simulink model "FMCWSim"  (R2021b)
settings: Solver=VariableStepAuto  StartTime=0.0  StopTime=stop_time  RelTol=1e-3
values from neighbouring files (symbols this model uses):
  num_samples_in_sampling_period = obj.ADC_Samples    [Radar.m]
  num_samples_prior_to_sample_period = int32((obj.ADC_ValidStartTime_us + obj.IdleTime_us) *                 obj.ADC_SampleRate_MSps)    [Radar.m]
  simulator = Simulator_revB()    [compute_sensed_targets.m]    (also in compute_sensed_values.m)
undefined symbols (not defined in the file or in its folder): designMultirateFIR, magnitude, physconst
libraries: phaseddetectlib x5, phasedenvlib x4, hdlsllib x4, simulink x2, phasedtxrxlib x2, phasedwavlib x1, dspswit3 x1, radarlib x1, dspmlti4 x1
settings Model: SimulationMode=accelerator  Creator=David  LastModifiedBy=David

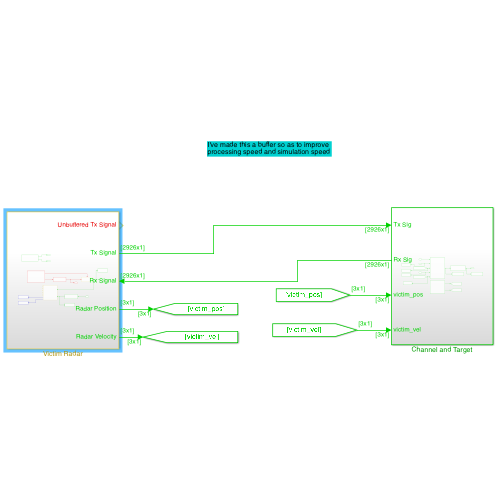
[thumbnail: Simulink's stored preview of the top-level diagram]
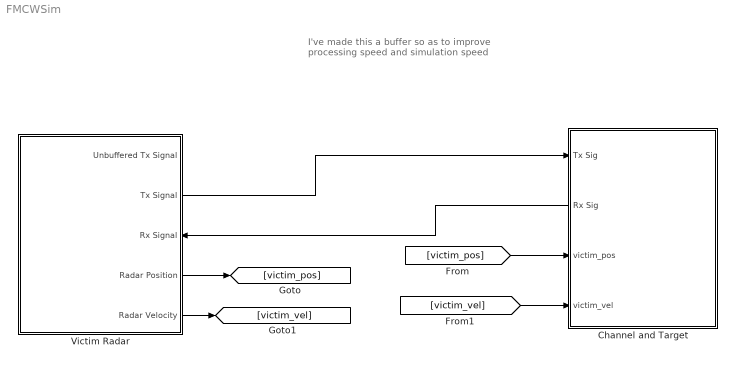
== system FMCWSim ==
  note: I've made this a buffer so as to improve
      | processing speed and simulation speed
  Channel and Target : Subsystem
      settings: PortSchema="{\"entries\":[{\"content\":{\"sides\":[{\"content\":{\"connectorIds\":[\"In1\",\"Out1\",\"In2\",\"In3\"]},\"type\":\"ConnectorPlacement.EquallySpacedRectSide\",\"uuid\":\"8c997438-cd57-4b9a-9eea-b04952771858\"},{\"content\":{\"connectorIds\":[],\"side\":\"RIGHT\"},\"type\":\"ConnectorPlacement.EquallySpacedRectSide\",\"uuid\":\"a5c22adb-228f-478b-86ad-e927dc02fa6c\"},{\"content\":{\"connectorIds\":[],\"side\":\"TOP\"},\"type\":\"ConnectorPlacement.EquallySpacedRectSide\",\"uuid\":\"b1cfcadd-6889-4e9e-8c43-7e76de170b82\"}]},\"type\":\"ConnectorPlacement.EquallySpacedConnector\",\"uuid\":\"fd8de1ec-06fb-4ea8-b936-70a4a20a8787\"}],\"packageUris\":[\"http://schema.mathworks.com/mf0/Connector/R2020b\"],\"version\":\"1.0\"}"
  Victim Radar : Subsystem
      settings: PortSchema="{\"entries\":[{\"content\":{\"sides\":[{\"content\":{\"connectorIds\":[]},\"type\":\"ConnectorPlacement.EquallySpacedRectSide\",\"uuid\":\"d1da3d36-0806-43d7-8452-bab3645a751c\"},{\"content\":{\"connectorIds\":[\"Out1\",\"Out2\",\"In1\",\"Out3\",\"Out4\"],\"side\":\"RIGHT\"},\"type\":\"ConnectorPlacement.EquallySpacedRectSide\",\"uuid\":\"352ec7eb-fc0a-43de-8b0c-663d6e923176\"},{\"content\":{\"connectorIds\":[],\"side\":\"TOP\"},\"type\":\"ConnectorPlacement.EquallySpacedRectSide\",\"uuid\":\"55e1007f-228b-4090-badb-c8b9047c2b51\"}]},\"type\":\"ConnectorPlacement.EquallySpacedConnector\",\"uuid\":\"2018d0fb-49bb-41d2-bc14-1588bf842768\"}],\"packageUris\":[\"http://schema.mathworks.com/mf0/Connector/R2020b\"],\"version\":\"1.0\"}"
  wires:
  [victim_pos] -> Channel and Target/2(victim_pos)
  [victim_vel] -> Channel and Target/3(victim_vel)
  Victim Radar/2(Tx Signal) -> Channel and Target/1(Tx Sig)
  Victim Radar/4(Radar Velocity) -> [victim_vel]
  Victim Radar/3(Radar Position) -> [victim_pos]
  Channel and Target/1(Rx Sig) -> Victim Radar/1(Rx Signal)

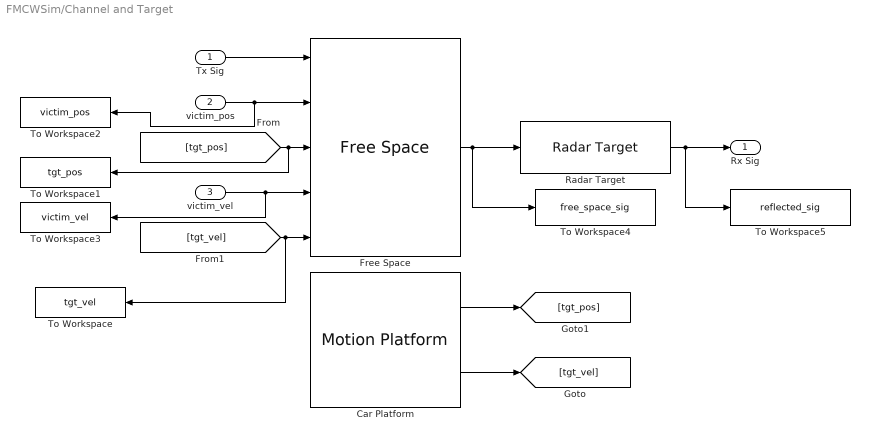
== system FMCWSim/Channel and Target ==
  Tx Sig : Inport
  victim_pos : Inport  Port=2
  victim_vel : Inport  Port=3
  Car Platform : phasedenvlib/Motion Platform  MotionModel=Velocity  InitialPosition=simulator.SimulatedTarget.position_m  InitialVelocity=[ 0; 0; 0 ]  VelocitySource=Property  Velocity=simulator.SimulatedTarget.velocity_meters_per_s  AccelerationSource=Property  Acceleration=[0;0;0]  CustomTrajectory=[ 0, 0, 0, 0, 0, 0, 0; 1, 0, 0, 0, 0, 0, 0 ]  ScanMode=None  InitialScanAngle=0  AzimuthSpan=[ -60, 60 ]  AzimuthScanRate=10  InitialOrientationAxes=eye( 3 )  OrientationAxesOutputPort=off  ElapsedTimeSource=Auto  SampleRateFromInputCheckbox=on  SampleRate=1e6  SimulateUsing=Interpreted execution
      settings: SourceProductBaseCode=AR
  Free Space : phasedenvlib/Free Space  PropagationSpeed=physconst( 'LightSpeed' )  OperatingFrequency=simulator.SimulatedTarget.operating_frequency_Hz  TwoWayPropagation=on  SampleRateFromInputCheckbox=off  SampleRate=simulator.Victim.FMCW_sampling_rate_Hz  MaximumDistanceSource=Property  MaximumDistance=1e3  MaximumNumInputSamplesSource=Auto  MaximumNumInputSamples=1000  SimulateUsing=Interpreted execution
      settings: SourceProductBaseCode=AR
  Radar Target : phasedenvlib/Radar Target  EnablePolarization=off  Mode=Monostatic  MeanRCSSource=Property  ScatteringMatrixSource=Property  MeanRCS=simulator.SimulatedTarget.rcs_sq_meters  ScatteringMatrix=eye( 2 )  Model=Nonfluctuating  PropagationSpeed=physconst( 'LightSpeed' )  OperatingFrequency=simulator.SimulatedTarget.operating_frequency_Hz  SeedSource=Auto  Seed=0  SimulateUsing=Interpreted execution
      settings: SourceProductBaseCode=AR
  To Workspace : ToWorkspace  VariableName=tgt_vel  SampleTime=-1
      settings: MaxDataPoints=2
  To Workspace1 : ToWorkspace  VariableName=tgt_pos  SampleTime=-1
      settings: MaxDataPoints=2
  To Workspace2 : ToWorkspace  VariableName=victim_pos  SampleTime=-1
      settings: MaxDataPoints=2
  To Workspace3 : ToWorkspace  VariableName=victim_vel  SampleTime=-1
      settings: MaxDataPoints=2
  To Workspace4 : ToWorkspace  VariableName=free_space_sig  SampleTime=-1
      settings: MaxDataPoints=2
  To Workspace5 : ToWorkspace  VariableName=reflected_sig  SampleTime=-1
      settings: MaxDataPoints=2
  Rx Sig : Outport
  wires:
  Tx Sig/1 -> Free Space/1
  victim_pos/1 -> To Workspace2/1, Free Space/2
  victim_vel/1 -> To Workspace3/1, Free Space/4
  [tgt_vel] -> To Workspace/1, Free Space/5
  [tgt_pos] -> To Workspace1/1, Free Space/3
  Car Platform/1 -> [tgt_pos]
  Car Platform/2 -> [tgt_vel]
  Radar Target/1 -> To Workspace5/1, Rx Sig/1
  Free Space/1 -> To Workspace4/1, Radar Target/1

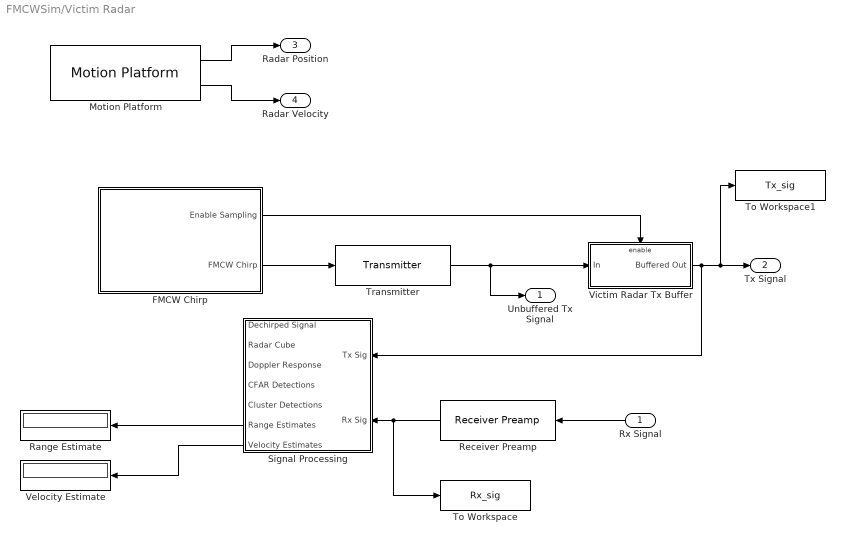
== system FMCWSim/Victim Radar ==
  Rx Signal : Inport
  FMCW Chirp : Subsystem
  Motion Platform : phasedenvlib/Motion Platform  MotionModel=Velocity  InitialPosition=simulator.Victim.position_m  InitialVelocity=[ 0; 0; 0 ]  VelocitySource=Property  Velocity=simulator.Victim.velocity_m_per_s  AccelerationSource=Property  Acceleration=[0;0;0]  CustomTrajectory=[ 0, 0, 0, 0, 0, 0, 0; 1, 0, 0, 0, 0, 0, 0 ]  ScanMode=None  InitialScanAngle=0  AzimuthSpan=[ -60, 60 ]  AzimuthScanRate=10  InitialOrientationAxes=eye( 3 )  OrientationAxesOutputPort=off  ElapsedTimeSource=Auto  SampleRateFromInputCheckbox=on  SampleRate=1e6  SimulateUsing=Interpreted execution
      settings: SourceProductBaseCode=AR
  Range Estimate : Display
  Receiver Preamp : phasedtxrxlib/Receiver Preamp  Gain=simulator.Victim.rx_gain_dB  LossFactor=0  NoiseMethod=Noise temperature  NoiseFigure=simulator.Victim.rx_nf_dB  ReferenceTemperature=290  SampleRateFromInputCheckbox=off  SampleRate=simulator.Victim.FMCW_sampling_rate_Hz  NoisePower=0  EnableInputPort=off  PhaseNoiseInputPort=off  SeedSource=Auto  Seed=0  SimulateUsing=Interpreted execution
      settings: SourceProductBaseCode=AR
  Signal Processing : Subsystem
  To Workspace : ToWorkspace  VariableName=Rx_sig  SampleTime=-1
      settings: MaxDataPoints=2
  To Workspace1 : ToWorkspace  VariableName=Tx_sig  SampleTime=-1
      settings: MaxDataPoints=2
  Transmitter : phasedtxrxlib/Transmitter  PeakPower=simulator.Victim.tx_power_W  Gain=simulator.Victim.tx_gain_dB  LossFactor=0  InUseOutputPort=off  CoherentOnTransmit=on  PhaseNoiseOutputPort=off  SeedSource=Auto  Seed=0  SimulateUsing=Interpreted execution
      settings: SourceProductBaseCode=AR
  Velocity Estimate : Display
  Victim Radar Tx Buffer : Subsystem  TreatAsAtomicUnit=on
  Unbuffered Tx Signal : Outport
  Tx Signal : Outport  Port=2
  Radar Position : Outport  Port=3
  Radar Velocity : Outport  Port=4
  wires:
  Rx Signal/1 -> Receiver Preamp/1
  Receiver Preamp/1 -> To Workspace/1, Signal Processing/2(Rx Sig)
  Signal Processing/6(Range Estimates) -> Range Estimate/1
  Signal Processing/7(Velocity Estimates) -> Velocity Estimate/1
  Motion Platform/2 -> Radar Velocity/1
  Motion Platform/1 -> Radar Position/1
  FMCW Chirp/2(FMCW Chirp) -> Transmitter/1
  FMCW Chirp/1(Enable Sampling) -> Victim Radar Tx Buffer/Enable
  Transmitter/1 -> Unbuffered Tx Signal/1, Victim Radar Tx Buffer/1(In)
  Victim Radar Tx Buffer/1(Buffered Out) -> To Workspace1/1, Tx Signal/1, Signal Processing/1(Tx Sig)

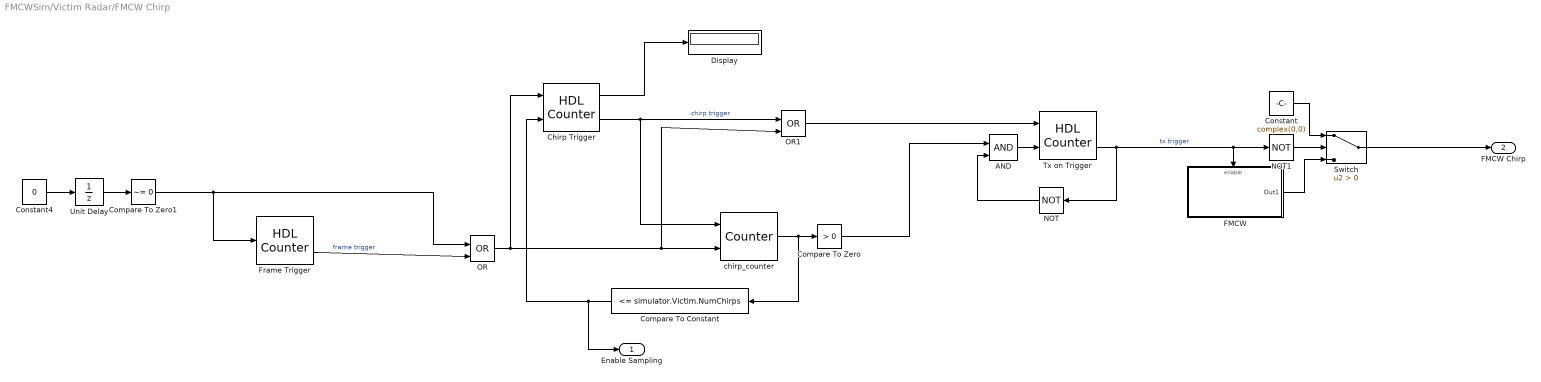
== system FMCWSim/Victim Radar/FMCW Chirp ==
  AND : Logic  IconShape=distinctive  AllPortsSameDT=off  OutDataTypeStr=boolean
  Chirp Trigger : hdlsllib/Sources/HDL Counter  CountType=Count limited  CountInit=1  CountStep=1  CountMax=simulator.Victim.FMCW_sampling_rate_Hz * simulator.Victim.sweep_time + simulator.Victim.num_samples_idle_time  CountFromType=Initial value  CountFrom=1  CountResetPort=on  CountLoadPort=off  CountEnbPort=on  CountDirPort=off  CountHitOutputPort=on  CountDataType=Unsigned  CountWordLen=16  CountFracLen=0  CountSampTime=1
  Compare To Constant : simulink/Logic and Bit Operations/Compare To Constant  relop=<=  const=simulator.Victim.NumChirps  OutDataTypeStr=boolean
  Compare To Zero : hdlsllib/Logic and Bit Operations/Compare To Zero  relop=>  OutDataTypeStr=boolean
      settings: SourceProductBaseCode=SL
  Compare To Zero1 : simulink/Logic and Bit Operations/Compare To Zero  relop=~=  OutDataTypeStr=boolean
  Constant : Constant  Value=complex(0,0)
  Constant4 : Constant  Value=0
  Display : Display
  FMCW : Subsystem
  Frame Trigger : hdlsllib/Sources/HDL Counter  CountType=Count limited  CountInit=1  CountStep=1  CountMax=simulator.Victim.num_samples_per_frame  CountFromType=Initial value  CountFrom=1  CountResetPort=on  CountLoadPort=off  CountEnbPort=off  CountDirPort=off  CountHitOutputPort=on  CountDataType=Unsigned  CountWordLen=32  CountFracLen=0  CountSampTime=1
  NOT : Logic  Operator=NOT  IconShape=distinctive  AllPortsSameDT=off  OutDataTypeStr=boolean
  NOT1 : Logic  Operator=NOT  IconShape=distinctive  AllPortsSameDT=off  OutDataTypeStr=boolean
  OR : Logic  Operator=OR  IconShape=distinctive  AllPortsSameDT=off  OutDataTypeStr=boolean
  OR1 : Logic  Operator=OR  IconShape=distinctive  AllPortsSameDT=off  OutDataTypeStr=boolean
  Switch : Switch  Criteria=u2 > Threshold
  Tx on Trigger : hdlsllib/Sources/HDL Counter  CountType=Count limited  CountInit=1  CountStep=1  CountMax=simulator.Victim.num_samples_idle_time  CountFromType=Initial value  CountFrom=1  CountResetPort=on  CountLoadPort=off  CountEnbPort=on  CountDirPort=off  CountHitOutputPort=on  CountDataType=Unsigned  CountWordLen=16  CountFracLen=0  CountSampTime=1
  Unit Delay : UnitDelay  InitialCondition=1  SampleTime=-1  HasFrameUpgradeWarning=on
  chirp_counter : dspswit3/Counter  Direction=Up  CountEvent=Rising edge  CounterSize=User defined  MaxCount=simulator.Victim.NumChirps + 1  InitialCount=1  Output=Count  HitValue=32  ResetInput=on  SamplesPerFrame=1  Ts=1  CntDtype=int16  HitDtype=Logical
  Enable Sampling : Outport
  FMCW Chirp : Outport  Port=2
  wires:
  Switch/1 -> FMCW Chirp/1
  chirp_counter/1 -> Compare To Constant/1, Compare To Zero/1
  Tx on Trigger/2 -> NOT/1, FMCW/Enable, NOT1/1  "tx trigger"
  AND/1 -> Tx on Trigger/2
  FMCW/1(Out1) -> Switch/3
  NOT1/1 -> Switch/2
  Constant/1 -> Switch/1
  Chirp Trigger/2 -> chirp_counter/1, OR1/1  "chirp trigger"
  Compare To Zero/1 -> AND/1
  NOT/1 -> AND/2
  Compare To Constant/1 -> Enable Sampling/1, Chirp Trigger/2
  Frame Trigger/2 -> OR/2  "frame trigger"
  Compare To Zero1/1 -> Frame Trigger/1, OR/1
  OR/1 -> Chirp Trigger/1, OR1/2, chirp_counter/2
  OR1/1 -> Tx on Trigger/1
  Unit Delay/1 -> Compare To Zero1/1
  Constant4/1 -> Unit Delay/1
  Chirp Trigger/1 -> Display/1

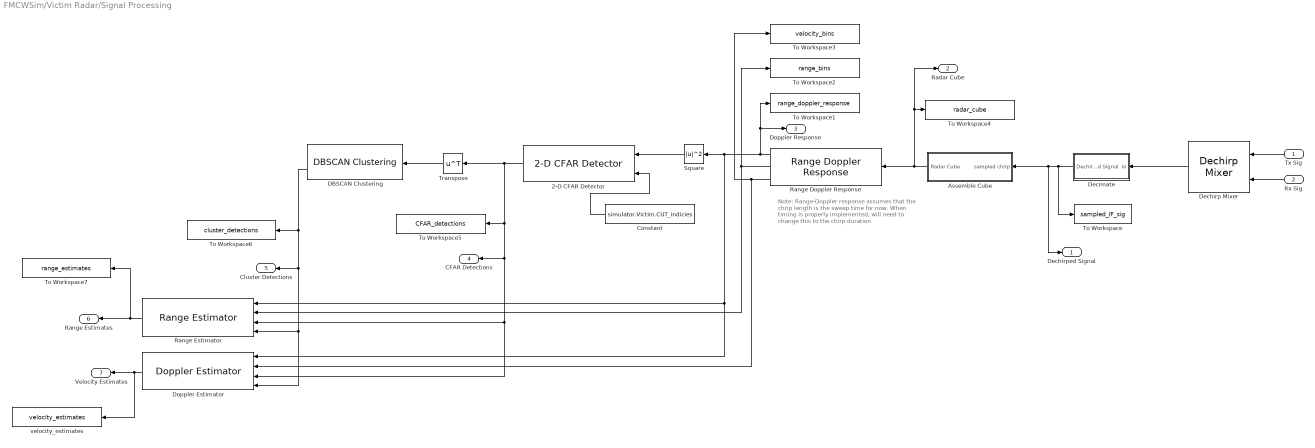
== system FMCWSim/Victim Radar/Signal Processing ==
  note: Note: Range-Doppler response assumes
      | that the chrip length is the sweep time
      | for now. When timing is properly implemented,
      | will need to change this to the chirp duration
  Tx Sig : Inport
  Rx Sig : Inport  Port=2
  2-D CFAR Detector : phaseddetectlib/2-D CFAR Detector  Method=CA  Rank=1  GuardBandSize=simulator.Victim.guard_region  TrainingBandSize=simulator.Victim.training_region  ThresholdFactor=Auto  ProbabilityFalseAlarm=simulator.Victim.PFAR  CustomThresholdFactor=1  OutputFormat=Detection index  ThresholdOutputPort=off  NoisePowerOutputPort=off  NumDetectionsSource=Auto  NumDetections=1  SimulateUsing=Interpreted execution
      settings: SourceProductBaseCode=AR
  Assemble Cube : Subsystem
  Constant : Constant  Value=simulator.Victim.CUT_indicies  VectorParams1D=off
  DBSCAN Clustering : radarlib/DBSCAN Clustering  BlockOutputs=Index and Cluster ID  EpsilonSource=Property  Epsilon=2  MinNumPoints=3  MaxNumPoints=10  EpsilonHistoryLength=10  EnableDisambiguation=off  AmbiguousDimension=1  SimulateUsing=Interpreted execution
      settings: SourceProductBaseCode=RA
  Dechirp Mixer : phaseddetectlib/Dechirp Mixer
      settings: SourceProductBaseCode=AR
  Decimate : Subsystem
  Doppler Estimator : phaseddetectlib/Doppler Estimator  NumEstimatesSource=Property  NumEstimates=5  VarianceOutputPort=off  NumPulses=2  NoisePowerSource=Property  NoisePower=1  ClusterInputPort=on  SimulateUsing=Interpreted execution
      settings: SourceProductBaseCode=AR
  Range Doppler Response : phaseddetectlib/Range Doppler Response  RangeMethod=FFT  PropagationSpeed=physconst( 'lightspeed' )  SampleRateFromInputCheckbox=off  SampleRate=simulator.Victim.ADC_SampleRate_MSps * 1e6  SweepSlope=simulator.Victim.FrequencySlope_MHz_us * 1e12  DechirpInput=off  RangeFFTLengthSource=Auto  RangeFFTLength=1024  RangeWindow=Hann  RangeSidelobeAttenuation=30  CustomRangeWindow=@hamming  ReferenceRangeCentered=off  ReferenceRange=0  MaximumNumInputSamplesSource=Auto  MaximumNumInputSamples=100  PRFSource=Property  PRF=1 / (simulator.Victim.ChirpCycleTime_us *1e6)  DopplerFFTLengthSource=Property  DopplerFFTLength=simulator.Victim.NumChirps  DopplerWindow=Hann  DopplerSidelobeAttenuation=30  CustomDopplerWindow=@hamming  DopplerOutput=Speed  OperatingFrequency=simulator.Victim.StartFrequency_GHz * 1e9  SimulateUsing=Code generation
      settings: SourceProductBaseCode=AR
  Range Estimator : phaseddetectlib/Range Estimator  NumEstimatesSource=Property  NumEstimates=5  VarianceOutputPort=off  RMSResolution=1  NoisePowerSource=Property  NoisePower=1  ClusterInputPort=on  SimulateUsing=Interpreted execution
      settings: SourceProductBaseCode=AR
  Square : Math  Operator=magnitude^2  SaturateOnIntegerOverflow=on
  To Workspace : ToWorkspace  VariableName=sampled_IF_sig  SampleTime=-1
      settings: MaxDataPoints=2
  To Workspace1 : ToWorkspace  VariableName=range_doppler_response  SampleTime=-1
      settings: MaxDataPoints=1
  To Workspace2 : ToWorkspace  VariableName=range_bins  SampleTime=-1
      settings: MaxDataPoints=1
  To Workspace3 : ToWorkspace  VariableName=velocity_bins  SampleTime=-1
      settings: MaxDataPoints=1
  To Workspace4 : ToWorkspace  VariableName=radar_cube  SampleTime=-1
      settings: MaxDataPoints=1
  To Workspace5 : ToWorkspace  VariableName=CFAR_detections  SampleTime=-1
      settings: MaxDataPoints=1
  To Workspace6 : ToWorkspace  VariableName=cluster_detections  SampleTime=-1
      settings: MaxDataPoints=1
  To Workspace7 : ToWorkspace  VariableName=range_estimates  SampleTime=-1
      settings: MaxDataPoints=1
  Transpose : Math  Operator=transpose  SaturateOnIntegerOverflow=on
  velocity_estimates : ToWorkspace  VariableName=velocity_estimates  SampleTime=-1
      settings: MaxDataPoints=1
  Dechirped Signal : Outport
  Radar Cube : Outport  Port=2
  Doppler Response : Outport  Port=3
  CFAR Detections : Outport  Port=4
  Cluster Detections : Outport  Port=5
  Range Estimates : Outport  Port=6
  Velocity Estimates : Outport  Port=7
  wires:
  Tx Sig/1 -> Dechirp Mixer/1
  Rx Sig/1 -> Dechirp Mixer/2
  Dechirp Mixer/1 -> Decimate/1(In)
  Decimate/1(Dechirped Signal) -> To Workspace/1, Dechirped Signal/1, Assemble Cube/1(sampled chirp)
  Assemble Cube/1(Radar Cube) -> Radar Cube/1, To Workspace4/1, Range Doppler Response/1
  Range Doppler Response/2 -> Range Estimator/2, To Workspace2/1
  Range Doppler Response/1 -> Doppler Estimator/1, Range Estimator/1, Square/1, Doppler Response/1, To Workspace1/1
  Range Doppler Response/3 -> Doppler Estimator/2, To Workspace3/1
  Square/1 -> 2-D CFAR Detector/1
  Constant/1 -> 2-D CFAR Detector/2
  2-D CFAR Detector/1 -> Transpose/1, Doppler Estimator/3, Range Estimator/3, CFAR Detections/1, To Workspace5/1
  DBSCAN Clustering/2 -> Doppler Estimator/4, Range Estimator/4, Cluster Detections/1, To Workspace6/1
  Transpose/1 -> DBSCAN Clustering/1
  Range Estimator/1 -> To Workspace7/1, Range Estimates/1
  Doppler Estimator/1 -> velocity_estimates/1, Velocity Estimates/1

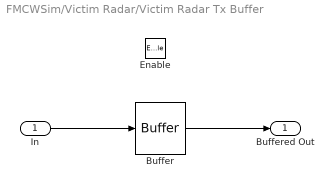
== system FMCWSim/Victim Radar/Victim Radar Tx Buffer ==
  In : Inport
  Enable : EnablePort
  Buffer : Buffer  N=int32(simulator.Victim.FMCW_sampling_rate_Hz * (simulator.Victim.sweep_time + simulator.Victim.IdleTime_us * 1e-6))  OutputFrames=off
  Buffered Out : Outport
  wires:
  In/1 -> Buffer/1
  Buffer/1 -> Buffered Out/1

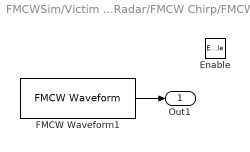
== system FMCWSim/Victim Radar/FMCW Chirp/FMCW ==
  Enable : EnablePort  StatesWhenEnabling=reset
  FMCW Waveform1 : phasedwavlib/FMCW Waveform  SampleRate=simulator.Victim.FMCW_sampling_rate_Hz  SweepTime=simulator.Victim.sweep_time  SweepBandwidth=simulator.Victim.Chirp_Tx_Bandwidth_MHz * 1e6  SweepDirection=Up  SweepInterval=Positive  OutputFormat=Samples  NumSamples=1  NumSweeps=waveform_params.num_sweeps  SimulateUsing=Interpreted execution
      settings: SourceProductBaseCode=AR
  Out1 : Outport
  wires:
  FMCW Waveform1/1 -> Out1/1

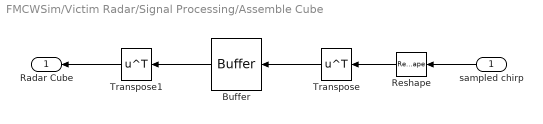
== system FMCWSim/Victim Radar/Signal Processing/Assemble Cube ==
  sampled chirp : Inport
  Buffer : Buffer  N=simulator.Victim.NumChirps  OutputFrames=off
  Reshape : Reshape
  Transpose : Math  Operator=transpose  SaturateOnIntegerOverflow=on
  Transpose1 : Math  Operator=transpose  SaturateOnIntegerOverflow=on
  Radar Cube : Outport
  wires:
  sampled chirp/1 -> Reshape/1
  Transpose/1 -> Buffer/1
  Buffer/1 -> Transpose1/1
  Transpose1/1 -> Radar Cube/1
  Reshape/1 -> Transpose/1

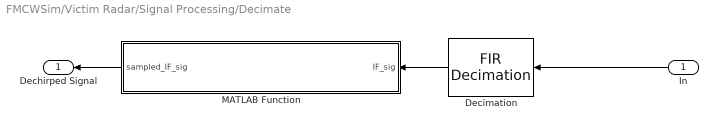
== system FMCWSim/Victim Radar/Signal Processing/Decimate ==
  In : Inport
  Decimation : dspmlti4/FIR Decimation  FilterSource=Auto  h=designMultirateFIR(1,2)  D=simulator.Victim.decimation_factor  filtStruct=Direct form  FilterObject=simulator.Victim.low_pass_filter  InputProcessing=Columns as channels (frame based)  framing=Enforce single-rate processing  inputOffset=0  outputBufInitCond=0  roundingMode=Floor  overflowMode=off  firstCoeffDataTypeStr=Inherit: Same word length as input  firstCoeffMin=[]  firstCoeffMax=[]  firstCoeffLastDataTypeStr=Inherit: Same word length as input  outputDataTypeStr=Inherit: Same as accumulator  outputMin=[]  outputMax=[]  outputLastDataTypeStr=Inherit: Same as accumulator
  MATLAB Function : MATLAB Function  TreatAsAtomicUnit=on
  Dechirped Signal : Outport
  wires:
  Decimation/1 -> MATLAB Function/1(IF_sig)
  MATLAB Function/1(sampled_IF_sig) -> Dechirped Signal/1
  In/1 -> Decimation/1

== matlab function FMCWSim/Victim Radar/Signal Processing/Decimate/MATLAB Function ==
  data: IF_sig input; sampled_IF_sig output; num_samples_prior_to_sample_period parameter; num_samples_in_sampling_period parameter
function sampled_IF_sig = select_sampled_IF_sig(IF_sig,num_samples_prior_to_sample_period,num_samples_in_sampling_period)

    sampled_IF_sig = IF_sig(...
        num_samples_prior_to_sample_period + 1:...
        num_samples_prior_to_sample_period + num_samples_in_sampling_period);
